simulink library "Atmosphere"  (R2024a)
settings: Solver=VariableStepAuto  StartTime=0.0  StopTime=10.0  RelTol=1e-3
settings Model: Creator=mahariansyah  LastModifiedBy=mahariansyah

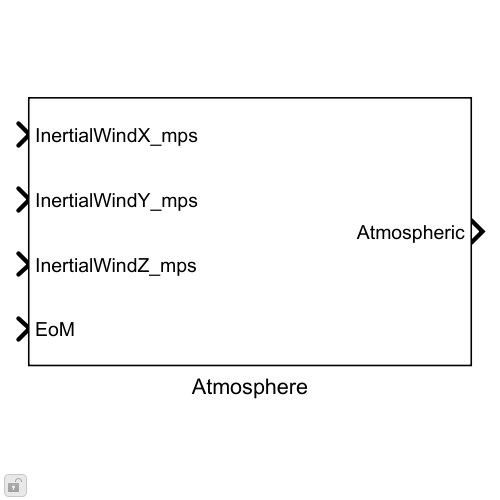
[thumbnail: Simulink's stored preview of the top-level diagram]
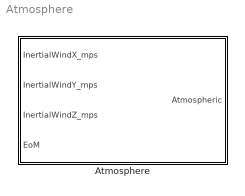
== system Atmosphere ==
  Atmosphere : Subsystem

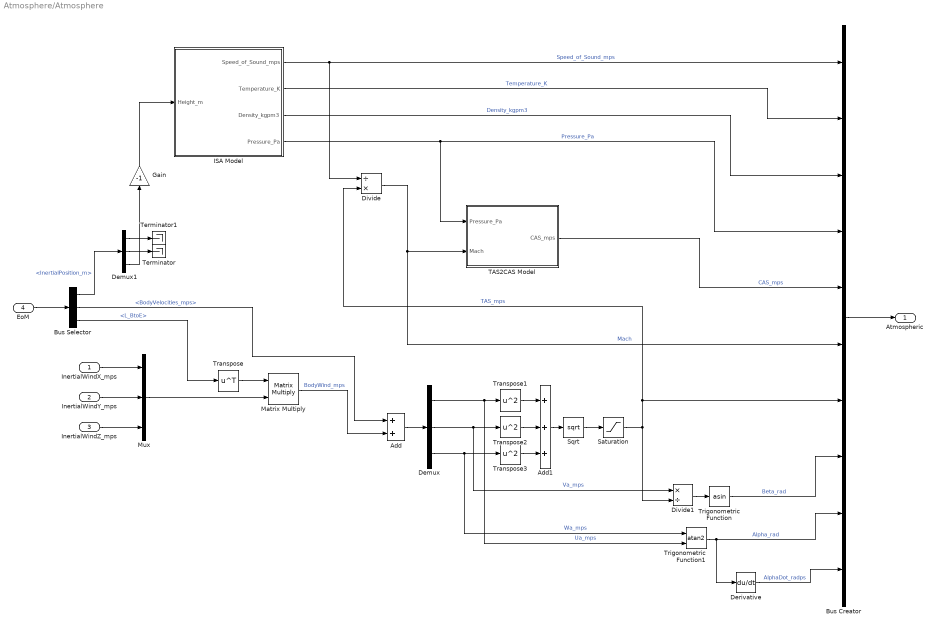
== system Atmosphere/Atmosphere ==
  InertialWindX_mps : Inport
  InertialWindY_mps : Inport  Port=2
  InertialWindZ_mps : Inport  Port=3
  EoM : Inport  Port=4
  Add : Sum
  Add1 : Sum  Inputs=+++
  Bus Creator : BusCreator  Inputs=10
  Bus Selector : BusSelector  OutputSignals=InertialPosition_m,BodyVelocities_mps,L_BtoE
  Demux : Demux  Outputs=3
  Demux1 : Demux  Outputs=3
  Derivative : Derivative
  Divide : Product  Inputs=/*
  Divide1 : Product  Inputs=*/
  Gain : Gain  Gain=-1
  ISA Model : Subsystem
  Matrix Multiply : Product  Multiplication=Matrix(*)
  Mux : Mux  Inputs=3
  Saturation : Saturate  UpperLimit=inf  LowerLimit=0.1
  Sqrt : Sqrt
  TAS2CAS Model : Subsystem
  Terminator : Terminator
  Terminator1 : Terminator
  Transpose : Math  Operator=transpose
  Transpose1 : Math  Operator=square
  Transpose2 : Math  Operator=square
  Transpose3 : Math  Operator=square
  Trigonometric Function : Trigonometry  Operator=asin
  Trigonometric Function1 : Trigonometry  Operator=atan2
  Atmospheric : Outport
  wires:
  Saturation/1 -> Bus Creator/7, Divide/2, Divide1/2  "TAS_mps"
  Gain/1 -> ISA Model/1(Height_m)
  Demux1/2 -> Terminator/1
  Demux1/1 -> Terminator1/1
  Bus Selector/1 -> Demux1/1  "<InertialPosition_m>"
  Bus Selector/3 -> Transpose/1  "<L_BtoE>"
  Bus Selector/2 -> Add/1  "<BodyVelocities_mps>"
  ISA Model/2(Temperature_K) -> Bus Creator/2  "Temperature_K"
  Divide/1 -> Bus Creator/6, TAS2CAS Model/2(Mach)  "Mach"
  Trigonometric Function1/1 -> Bus Creator/9, Derivative/1  "Alpha_rad"
  InertialWindX_mps/1 -> Mux/1
  Transpose2/1 -> Add1/2
  Matrix Multiply/1 -> Add/2  "BodyWind_mps"
  Demux/1 -> Trigonometric Function1/2, Transpose1/1  "Ua_mps"
  Transpose1/1 -> Add1/1
  Demux/3 -> Trigonometric Function1/1, Transpose3/1  "Wa_mps"
  InertialWindZ_mps/1 -> Mux/3
  Add/1 -> Demux/1
  Trigonometric Function/1 -> Bus Creator/8  "Beta_rad"
  ISA Model/3(Density_kgpm3) -> Bus Creator/3  "Density_kgpm3"
  Transpose3/1 -> Add1/3
  Sqrt/1 -> Saturation/1
  Demux/2 -> Transpose2/1, Divide1/1  "Va_mps"
  ISA Model/4(Pressure_Pa) -> Bus Creator/4, TAS2CAS Model/1(Pressure_Pa)  "Pressure_Pa"
  EoM/1 -> Bus Selector/1
  InertialWindY_mps/1 -> Mux/2
  Add1/1 -> Sqrt/1
  Transpose/1 -> Matrix Multiply/1
  Demux1/3 -> Gain/1
  Mux/1 -> Matrix Multiply/2
  ISA Model/1(Speed_of_Sound_mps) -> Bus Creator/1, Divide/1  "Speed_of_Sound_mps"
  Bus Creator/1 -> Atmospheric/1
  Divide1/1 -> Trigonometric Function/1
  Derivative/1 -> Bus Creator/10  "AlphaDot_radps"
  TAS2CAS Model/1(CAS_mps) -> Bus Creator/5  "CAS_mps"

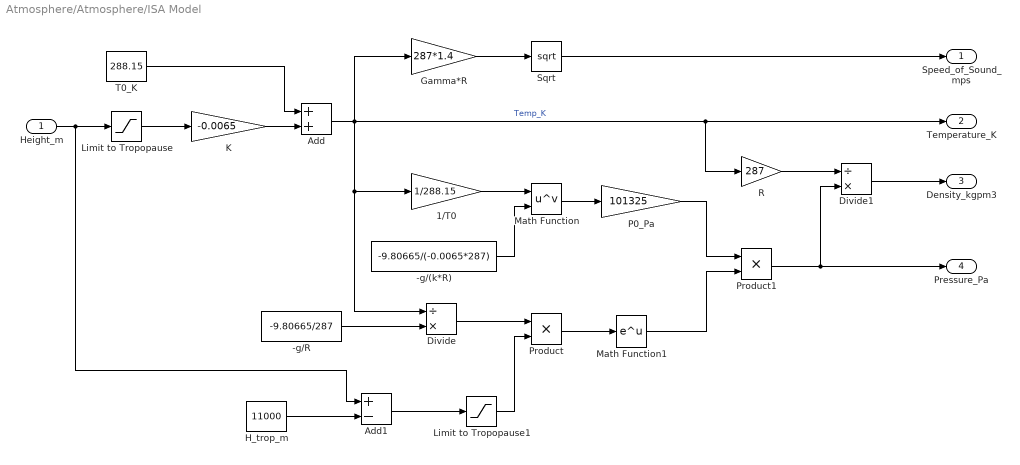
== system Atmosphere/Atmosphere/ISA Model ==
  Height_m : Inport
  -g/(k*R) : Constant  Value=-9.80665/(-0.0065*287)
  -g/R : Constant  Value=-9.80665/287
  1/T0 : Gain  Gain=1/288.15
  Add : Sum
  Add1 : Sum  Inputs=+-
  Divide : Product  Inputs=/*
  Divide1 : Product  Inputs=/*
  Gamma*R : Gain  Gain=287*1.4
  H_trop_m : Constant  Value=11000
  K : Gain  Gain=-0.0065
  Limit to Tropopause : Saturate  UpperLimit=11000  LowerLimit=0
  Limit to Tropopause1 : Saturate  UpperLimit=inf  LowerLimit=0
  Math Function : Math  Operator=pow
  Math Function1 : Math
  P0_Pa : Gain  Gain=101325
  Product : Product
  Product1 : Product
  R : Gain  Gain=287
  Sqrt : Sqrt
  T0_K : Constant  Value=288.15
  Speed_of_Sound_mps : Outport
  Temperature_K : Outport  Port=2
  Density_kgpm3 : Outport  Port=3
  Pressure_Pa : Outport  Port=4
  wires:
  Add/1 -> Gamma*R/1, Temperature_K/1, R/1, 1/T0/1, Divide/1  "Temp_K"
  Limit to Tropopause/1 -> K/1
  Add1/1 -> Limit to Tropopause1/1
  Math Function1/1 -> Product1/2
  Product1/1 -> Pressure_Pa/1, Divide1/2
  Divide/1 -> Product/1
  Math Function/1 -> P0_Pa/1
  P0_Pa/1 -> Product1/1
  Sqrt/1 -> Speed_of_Sound_mps/1
  Height_m/1 -> Add1/1, Limit to Tropopause/1
  Limit to Tropopause1/1 -> Product/2
  K/1 -> Add/2
  T0_K/1 -> Add/1
  Gamma*R/1 -> Sqrt/1
  H_trop_m/1 -> Add1/2
  -g/R/1 -> Divide/2
  -g/(k*R)/1 -> Math Function/2
  R/1 -> Divide1/1
  1/T0/1 -> Math Function/1
  Divide1/1 -> Density_kgpm3/1
  Product/1 -> Math Function1/1

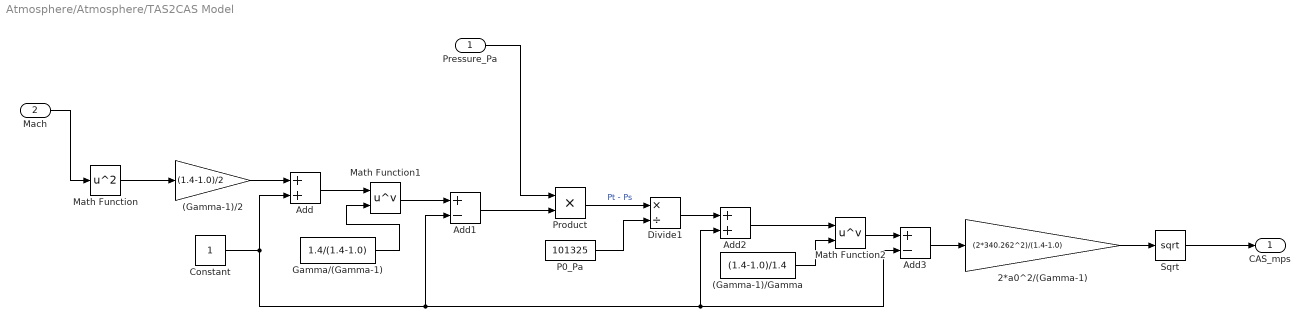
== system Atmosphere/Atmosphere/TAS2CAS Model ==
  Pressure_Pa : Inport
  Mach : Inport  Port=2
  (Gamma-1)/2 : Gain  Gain=(1.4-1.0)/2
  (Gamma-1)/Gamma : Constant  Value=(1.4-1.0)/1.4
  2*a0^2/(Gamma-1) : Gain  Gain=(2*340.262^2)/(1.4-1.0)
  Add : Sum
  Add1 : Sum  Inputs=+-
  Add2 : Sum
  Add3 : Sum  Inputs=+-
  Constant : Constant
  Divide1 : Product  Inputs=*/
  Gamma/(Gamma-1) : Constant  Value=1.4/(1.4-1.0)
  Math Function : Math  Operator=square
  Math Function1 : Math  Operator=pow  SignedPower=on
  Math Function2 : Math  Operator=pow  SignedPower=on
  P0_Pa : Constant  Value=101325
  Product : Product
  Sqrt : Sqrt
  CAS_mps : Outport
  wires:
  Math Function1/1 -> Add1/1
  Gamma/(Gamma-1)/1 -> Math Function1/2
  P0_Pa/1 -> Divide1/2
  (Gamma-1)/2/1 -> Add/1
  Pressure_Pa/1 -> Product/1
  Add2/1 -> Math Function2/1
  (Gamma-1)/Gamma/1 -> Math Function2/2
  Math Function/1 -> (Gamma-1)/2/1
  Add1/1 -> Product/2
  Product/1 -> Divide1/1  "Pt - Ps"
  Mach/1 -> Math Function/1
  Constant/1 -> Add1/2, Add3/2, Add2/2, Add/2
  Math Function2/1 -> Add3/1
  Add/1 -> Math Function1/1
  Divide1/1 -> Add2/1
  2*a0^2/(Gamma-1)/1 -> Sqrt/1
  Add3/1 -> 2*a0^2/(Gamma-1)/1
  Sqrt/1 -> CAS_mps/1
